simulink model "test_induction_cooker_increasedecreasepower"  (R2022b)
settings: Solver=FixedStepAuto  StartTime=0.0  StopTime=120  FixedStep=0.1  RelTol=1e-3
settings Model: Creator=cristian  LastModifiedBy=cristian
settings ConfigComp: CovEnable=on  CovScope=ReferencedModels  CovIncludeTopModel=off  CovModelRefEnable=filtered

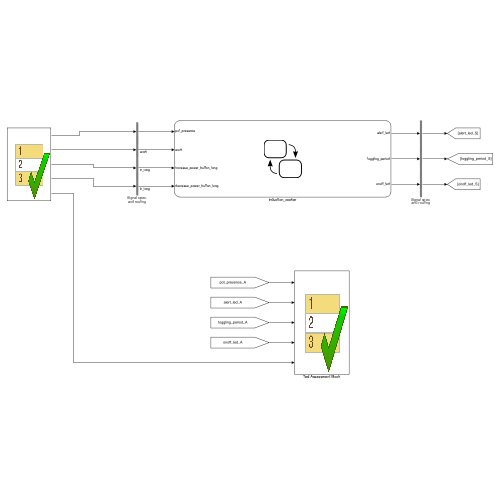
[thumbnail: Simulink's stored preview of the top-level diagram]
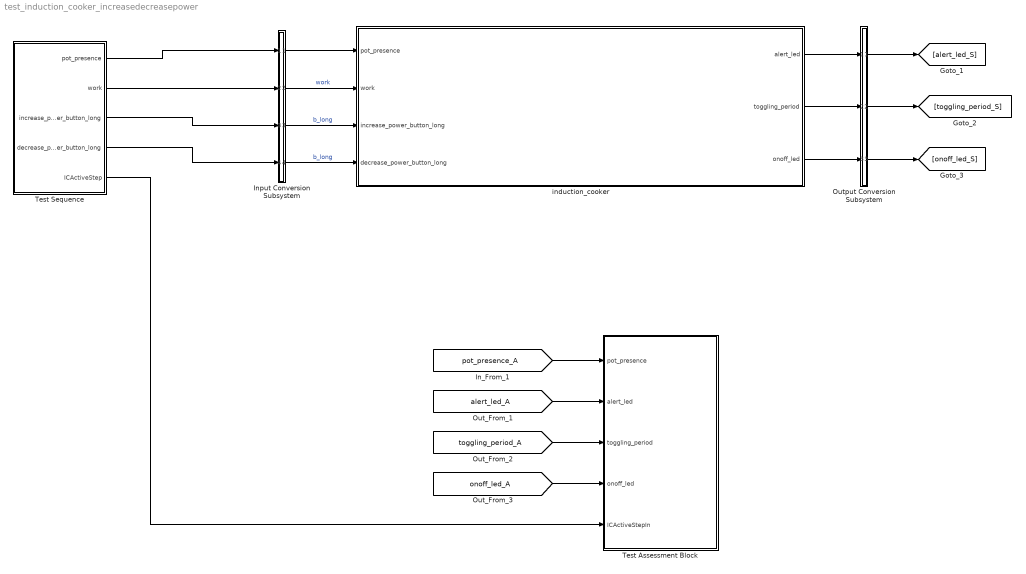
== system test_induction_cooker_increasedecreasepower ==
  Input Conversion Subsystem : Subsystem  Tag=__SLT_ICS__  Description=|
      | Signal spec.
      | and routing
      settings: AttributesFormatString=%<Description>
  Output Conversion Subsystem : Subsystem  Tag=__SLT_OCS__  Description=|
      | Signal spec.
      | and routing
      settings: AttributesFormatString=%<Description>
  Test Assessment Block : Test Sequence  Tag=__SLT_ASMT__  TreatAsAtomicUnit=on
  Test Sequence : Test Sequence  TreatAsAtomicUnit=on
  induction_cooker : Stateflow chart  TreatAsAtomicUnit=on
  wires:
  Test Sequence/1(pot_presence) -> Input Conversion Subsystem/1(Inport_1)
  Test Sequence/2(work) -> Input Conversion Subsystem/2(Inport_2)
  Test Sequence/3(increase_power_button_long) -> Input Conversion Subsystem/3(Inport_3)
  Test Sequence/4(decrease_power_button_long) -> Input Conversion Subsystem/4(Inport_4)
  Output Conversion Subsystem/1(Outport_1) -> [alert_led_S]
  Output Conversion Subsystem/2(Outport_2) -> [toggling_period_S]
  Output Conversion Subsystem/3(Outport_3) -> [onoff_led_S]
  Input Conversion Subsystem/1(Outport_1) -> induction_cooker/1(pot_presence)
  Input Conversion Subsystem/2(Outport_2) -> induction_cooker/2(work)  "work"
  Input Conversion Subsystem/3(Outport_3) -> induction_cooker/3(increase_power_button_long)  "b_long"
  Input Conversion Subsystem/4(Outport_4) -> induction_cooker/4(decrease_power_button_long)  "b_long"
  induction_cooker/1(alert_led) -> Output Conversion Subsystem/1(Inport_1)
  induction_cooker/2(toggling_period) -> Output Conversion Subsystem/2(Inport_2)
  induction_cooker/3(onoff_led) -> Output Conversion Subsystem/3(Inport_3)
  [onoff_led_A] -> Test Assessment Block/4(onoff_led)
  Test Sequence/5(ICActiveStep) -> Test Assessment Block/5(ICActiveStepIn)
  [toggling_period_A] -> Test Assessment Block/3(toggling_period)
  [alert_led_A] -> Test Assessment Block/2(alert_led)
  [pot_presence_A] -> Test Assessment Block/1(pot_presence)

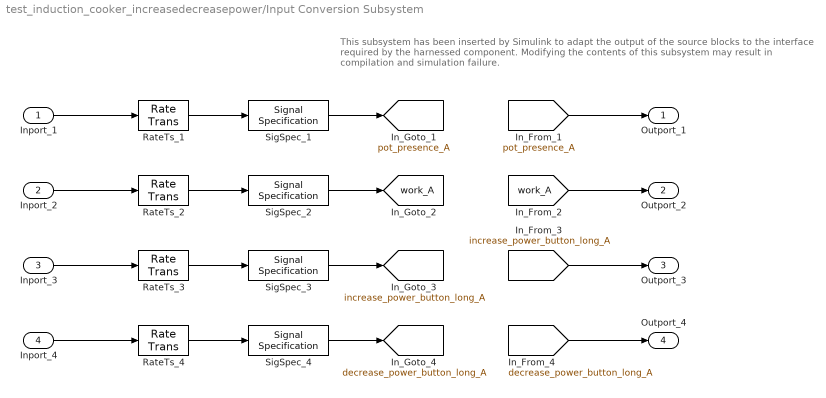
== system test_induction_cooker_increasedecreasepower/Input Conversion Subsystem ==
  note: This subsystem has been inserted by Simulink to adapt the output of the source blocks to the interface required by the harnessed component.
      |  Modifying the contents of this subsystem may result in compilation and simulation failure.
  Inport_1 : Inport
  Inport_2 : Inport  Port=2
  Inport_3 : Inport  Port=3
  Inport_4 : Inport  Port=4
  RateTs_1 : RateTransition  OutPortSampleTime=[-1, 0]
  RateTs_2 : RateTransition  OutPortSampleTime=[0, 1]
  RateTs_3 : RateTransition  OutPortSampleTime=[0, 1]
  RateTs_4 : RateTransition  OutPortSampleTime=[0, 1]
  SigSpec_1 : SignalSpecification  OutDataTypeStr=boolean  Dimensions=[1]  SampleTime=[-1, 0]
  SigSpec_2 : SignalSpecification  OutDataTypeStr=boolean  Dimensions=[1]  SampleTime=[0, 1]
  SigSpec_3 : SignalSpecification  OutDataTypeStr=boolean  Dimensions=[1]  SampleTime=[0, 1]
  SigSpec_4 : SignalSpecification  OutDataTypeStr=boolean  Dimensions=[1]  SampleTime=[0, 1]
  Outport_1 : Outport
  Outport_2 : Outport  Port=2
  Outport_3 : Outport  Port=3
  Outport_4 : Outport  Port=4
  tag scope: decrease_power_button_long_A=global, increase_power_button_long_A=global, pot_presence_A=global, work_A=global
  wires:
  [pot_presence_A] -> Outport_1/1
  SigSpec_1/1 -> [pot_presence_A]
  RateTs_1/1 -> SigSpec_1/1
  Inport_1/1 -> RateTs_1/1
  [work_A] -> Outport_2/1
  SigSpec_2/1 -> [work_A]
  RateTs_2/1 -> SigSpec_2/1
  Inport_2/1 -> RateTs_2/1
  [increase_power_button_long_A] -> Outport_3/1
  SigSpec_3/1 -> [increase_power_button_long_A]
  RateTs_3/1 -> SigSpec_3/1
  Inport_3/1 -> RateTs_3/1
  [decrease_power_button_long_A] -> Outport_4/1
  SigSpec_4/1 -> [decrease_power_button_long_A]
  RateTs_4/1 -> SigSpec_4/1
  Inport_4/1 -> RateTs_4/1

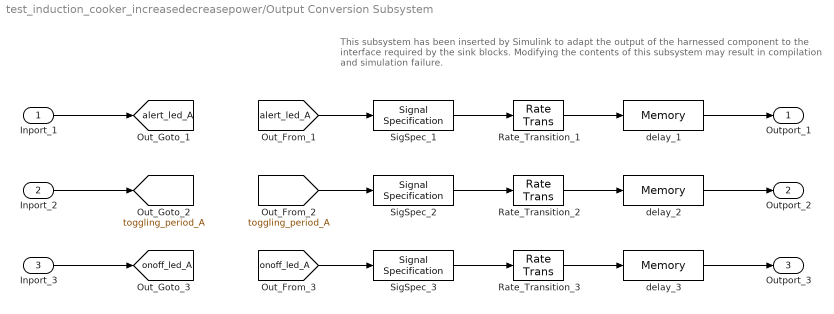
== system test_induction_cooker_increasedecreasepower/Output Conversion Subsystem ==
  note: This subsystem has been inserted by Simulink to adapt the output of the harnessed component to the interface required by the sink blocks.
      |  Modifying the contents of this subsystem may result in compilation and simulation failure.
  Inport_1 : Inport
  Inport_2 : Inport  Port=2
  Inport_3 : Inport  Port=3
  Rate_Transition_1 : RateTransition  OutPortSampleTimeOpt=Inherit
  Rate_Transition_2 : RateTransition  OutPortSampleTimeOpt=Inherit
  Rate_Transition_3 : RateTransition  OutPortSampleTimeOpt=Inherit
  SigSpec_1 : SignalSpecification  OutDataTypeStr=boolean  Dimensions=[1]
  SigSpec_2 : SignalSpecification  OutDataTypeStr=double  Dimensions=[1]
  SigSpec_3 : SignalSpecification  OutDataTypeStr=boolean  Dimensions=[1]
  delay_1 : Memory
  delay_2 : Memory
  delay_3 : Memory
  Outport_1 : Outport
  Outport_2 : Outport  Port=2
  Outport_3 : Outport  Port=3
  tag scope: alert_led_A=global, onoff_led_A=global, toggling_period_A=global
  wires:
  Inport_1/1 -> [alert_led_A]
  [alert_led_A] -> SigSpec_1/1
  SigSpec_1/1 -> Rate_Transition_1/1
  Rate_Transition_1/1 -> delay_1/1
  delay_1/1 -> Outport_1/1
  Inport_2/1 -> [toggling_period_A]
  [toggling_period_A] -> SigSpec_2/1
  SigSpec_2/1 -> Rate_Transition_2/1
  Rate_Transition_2/1 -> delay_2/1
  delay_2/1 -> Outport_2/1
  Inport_3/1 -> [onoff_led_A]
  [onoff_led_A] -> SigSpec_3/1
  SigSpec_3/1 -> Rate_Transition_3/1
  Rate_Transition_3/1 -> delay_3/1
  delay_3/1 -> Outport_3/1

== stateflow chart test_induction_cooker_increasedecreasepower/Test Assessment Block ==
  state IncreaseToMaxPower
    state step_1
      state Verify_IncreaseDecreasePower_Init
        verify(pot_presence == 0 && alert_led == 0 && abs(toggling_period - 0) < TOLERANCE && onoff_led == 0)
        settings: description=|
            | Inizializzazione.
            | Pentola presente, led di alert spento e potenza di erogazione nulla.
      state Verify_IncreaseDecreasePower_PowerOn
        verify(pot_presence == 0 && alert_led == 0 && abs(toggling_period - 0) < TOLERANCE && onoff_led == 1)
        settings: description=Richiesta di accensione del fornello.
      state Verify_IncreaseToMaxPower_PressFor300W
        verify(pot_presence == 0 && alert_led == 0 && abs(toggling_period - 0) < TOLERANCE && onoff_led == 1)
        settings: description=|
            | Pressione di richiesta incremento.
            | Pentola presente, led di alert spento e potenza di erogazione nulla.
            | Led di accensione acceso.
      state Verify_IncreaseToMaxPower_ReleaseFor300W
        verify(pot_presence == 0 && alert_led == 0 && abs(toggling_period - 0) < TOLERANCE && onoff_led == 1)
        settings: description=|
            | Rilascio bottone.
            | Pentola presente, led di alert spento e potenza di erogazione nulla.
            | Led di accensione acceso.
      state Verify_IncreaseToMaxPower_WaitIn300W
        verify(pot_presence == 0 && alert_led == 0 && abs(toggling_period - 2) < TOLERANCE && onoff_led == 1)
        settings: description=|
            | Stato di attesa di cambiamento potenza.
            | Pentola presente, led di alert spento e potenza di erogazione nulla.
            | Led di accensione acceso.
            | Frequenza di toggling incrementata.
      state Verify_IncreaseToMaxPower_PressFor500W
        verify(pot_presence == 0 && alert_led == 0 && abs(toggling_period - 2) < TOLERANCE && onoff_led == 1)
        settings: description=Pressione di richiesta incremento.
      state Verify_IncreaseToMaxPower_ReleaseFor500W
        verify(pot_presence == 0 && alert_led == 0 && abs(toggling_period - 2) < TOLERANCE && onoff_led == 1)
        settings: description=Rilascio bottone.
      state Verify_IncreaseToMaxPower_WaitIn500W
        verify(pot_presence == 0 && alert_led == 0 && abs(toggling_period - 1) < TOLERANCE && onoff_led == 1)
        settings: description=|
            | Stato di attesa di cambiamento potenza.
            | Pentola presente, led di alert spento e potenza di erogazione nulla.
            | Led di accensione acceso.
            | Frequenza di toggling incrementata.
      state Verify_IncreaseToMaxPower_PressFor1000W
        verify(pot_presence == 0 && alert_led == 0 && abs(toggling_period - 1) < TOLERANCE && onoff_led == 1)
        settings: description=Pressione di richiesta incremento.
      state Verify_IncreaseToMaxPower_ReleaseFor1000W
        verify(pot_presence == 0 && alert_led == 0 && abs(toggling_period - 1) < TOLERANCE && onoff_led == 1)
        settings: description=Rilascio bottone.
      state Verify_IncreaseToMaxPower_WaitIn1000W
        verify(pot_presence == 0 && alert_led == 0 && abs(toggling_period - 0.5) < TOLERANCE && onoff_led == 1)
        settings: description=|
            | Stato di attesa di cambiamento potenza.
            | Pentola presente, led di alert spento e potenza di erogazione nulla.
            | Led di accensione acceso.
            | Frequenza di toggling incrementata.
      state Verify_IncreaseToMaxPower_PressFor1500W
        verify(pot_presence == 0 && alert_led == 0 && abs(toggling_period - 0.5) < TOLERANCE && onoff_led == 1)
        settings: description=Pressione di richiesta incremento.
      state Verify_IncreaseToMaxPower_ReleaseFor1500W
        verify(pot_presence == 0 && alert_led == 0 && abs(toggling_period - 0.5) < TOLERANCE && onoff_led == 1)
        settings: description=Rilascio bottone.
      state Verify_IncreaseToMaxPower_WaitIn1500W
        verify(pot_presence == 0 && alert_led == 0 && abs(toggling_period - 0.25) < TOLERANCE && onoff_led == 1)
        settings: description=|
            | Stato di attesa di cambiamento potenza.
            | Pentola presente, led di alert spento e potenza di erogazione nulla.
            | Led di accensione acceso.
            | Frequenza di toggling incrementata.
      state Verify_DecreaseToMinPower_PressFor1000W
        verify(pot_presence == 0 && alert_led == 0 && abs(toggling_period - 0.25) < TOLERANCE && onoff_led == 1)
        settings: description=Pressione di richiesta decremento.
      state Verify_DecreaseToMinPower_ReleaseFor1000W
        verify(pot_presence == 0 && alert_led == 0 && abs(toggling_period - 0.25) < TOLERANCE && onoff_led == 1)
        settings: description=Rilascio bottone.
      state Verify_DecreaseToMinPower_WaitIn1000W
        verify(pot_presence == 0 && alert_led == 0 && abs(toggling_period - 0.50) < TOLERANCE && onoff_led == 1)
        settings: description=|
            | Stato di attesa di cambiamento potenza.
            | Pentola presente, led di alert spento e potenza di erogazione nulla.
            | Led di accensione acceso.
            | Frequenza di toggling decrementata.
      state Verify_DecreaseToMinPower_PressFor500W
        verify(pot_presence == 0 && alert_led == 0 && abs(toggling_period - 0.50) < TOLERANCE && onoff_led == 1)
        settings: description=Pressione di richiesta decremento.
      state Verify_DecreaseToMinPower_ReleaseFor500W
        verify(pot_presence == 0 && alert_led == 0 && abs(toggling_period - 0.50) < TOLERANCE && onoff_led == 1)
        settings: description=Rilascio bottone.
      state Verify_DecreaseToMinPower_WaitIn500W
        verify(pot_presence == 0 && alert_led == 0 && abs(toggling_period - 1) < TOLERANCE && onoff_led == 1)
        settings: description=|
            | Stato di attesa di cambiamento potenza.
            | Pentola presente, led di alert spento e potenza di erogazione nulla.
            | Led di accensione acceso.
            | Frequenza di toggling decrementata.
      state Verify_DecreaseToMinPower_PressFor300W
        verify(pot_presence == 0 && alert_led == 0 && abs(toggling_period - 1) < TOLERANCE && onoff_led == 1)
        settings: description=Pressione di richiesta decremento.
      state Verify_DecreaseToMinPower_ReleaseFor300W
        verify(pot_presence == 0 && alert_led == 0 && abs(toggling_period - 1) < TOLERANCE && onoff_led == 1)
        settings: description=Rilascio bottone.
      state Verify_DecreaseToMinPower_WaitIn300W
        verify(pot_presence == 0 && alert_led == 0 && abs(toggling_period - 2) < TOLERANCE && onoff_led == 1)
        settings: description=|
            | Stato di attesa di cambiamento potenza.
            | Pentola presente, led di alert spento e potenza di erogazione nulla.
            | Led di accensione acceso.
            | Frequenza di toggling decrementata.
      state step_1_1
      (default) -> (junction 238)
      step_1 -> (junction 238)
      (junction 238) -> (junction 239) [order 1] : [ICActiveStepIn == ICActiveStepEnum.IncreaseDecreasePower_Init
          | ]
      (junction 239) -> Verify_IncreaseDecreasePower_Init [order 1] : [~in(IncreaseToMaxPower.step_1.Verify_IncreaseDecreasePower_Init)]
      (junction 238) -> (junction 250) [order 2]
      (junction 239) -> (junction 242) [order 2]
      (junction 250) -> (junction 251) [order 1] : [ICActiveStepIn == ICActiveStepEnum.IncreaseDecreasePower_PowerOn
          | ]
      (junction 251) -> Verify_IncreaseDecreasePower_PowerOn [order 1] : [~in(IncreaseToMaxPower.step_1.Verify_IncreaseDecreasePower_PowerOn)]
      (junction 250) -> (junction 259) [order 2]
      (junction 251) -> (junction 254) [order 2]
      (junction 259) -> (junction 260) [order 1] : [ICActiveStepIn == ICActiveStepEnum.IncreaseToMaxPower_PressFor300W
          | ]
      (junction 260) -> Verify_IncreaseToMaxPower_PressFor300W [order 1] : [~in(IncreaseToMaxPower.step_1.Verify_IncreaseToMaxPower_PressFor300W)]
      (junction 259) -> (junction 268) [order 2]
      (junction 260) -> (junction 263) [order 2]
      (junction 268) -> (junction 269) [order 1] : [ICActiveStepIn == ICActiveStepEnum.IncreaseToMaxPower_ReleaseFor300W
          | ]
      (junction 269) -> Verify_IncreaseToMaxPower_ReleaseFor300W [order 1] : [~in(IncreaseToMaxPower.step_1.Verify_IncreaseToMaxPower_ReleaseFor300W)]
      (junction 268) -> (junction 277) [order 2]
      (junction 269) -> (junction 272) [order 2]
      (junction 277) -> (junction 278) [order 1] : [ICActiveStepIn == ICActiveStepEnum.IncreaseToMaxPower_WaitIn300W
          | ]
      (junction 278) -> Verify_IncreaseToMaxPower_WaitIn300W [order 1] : [~in(IncreaseToMaxPower.step_1.Verify_IncreaseToMaxPower_WaitIn300W)]
      (junction 277) -> (junction 286) [order 2]
      (junction 278) -> (junction 281) [order 2]
      (junction 286) -> (junction 287) [order 1] : [ICActiveStepIn == ICActiveStepEnum.IncreaseToMaxPower_PressFor500W
          | ]
      (junction 287) -> Verify_IncreaseToMaxPower_PressFor500W [order 1] : [~in(IncreaseToMaxPower.step_1.Verify_IncreaseToMaxPower_PressFor500W)]
      (junction 286) -> (junction 295) [order 2]
      (junction 287) -> (junction 290) [order 2]
      (junction 295) -> (junction 296) [order 1] : [ICActiveStepIn == ICActiveStepEnum.IncreaseToMaxPower_ReleaseFor500W
          | ]
      (junction 296) -> Verify_IncreaseToMaxPower_ReleaseFor500W [order 1] : [~in(IncreaseToMaxPower.step_1.Verify_IncreaseToMaxPower_ReleaseFor500W)]
      (junction 295) -> (junction 304) [order 2]
      (junction 296) -> (junction 299) [order 2]
      (junction 304) -> (junction 305) [order 1] : [ICActiveStepIn == ICActiveStepEnum.IncreaseToMaxPower_WaitIn500W
          | ]
      (junction 305) -> Verify_IncreaseToMaxPower_WaitIn500W [order 1] : [~in(IncreaseToMaxPower.step_1.Verify_IncreaseToMaxPower_WaitIn500W)]
      (junction 304) -> (junction 313) [order 2]
      (junction 305) -> (junction 308) [order 2]
      (junction 313) -> (junction 314) [order 1] : [ICActiveStepIn == ICActiveStepEnum.IncreaseToMaxPower_PressFor1000W
          | ]
      (junction 314) -> Verify_IncreaseToMaxPower_PressFor1000W [order 1] : [~in(IncreaseToMaxPower.step_1.Verify_IncreaseToMaxPower_PressFor1000W)]
      (junction 313) -> (junction 322) [order 2]
      (junction 314) -> (junction 317) [order 2]
      (junction 322) -> (junction 323) [order 1] : [ICActiveStepIn == ICActiveStepEnum.IncreaseToMaxPower_ReleaseFor1000W
          | ]
      (junction 323) -> Verify_IncreaseToMaxPower_ReleaseFor1000W [order 1] : [~in(IncreaseToMaxPower.step_1.Verify_IncreaseToMaxPower_ReleaseFor1000W)]
      (junction 322) -> (junction 331) [order 2]
      (junction 323) -> (junction 326) [order 2]
      (junction 331) -> (junction 332) [order 1] : [ICActiveStepIn == ICActiveStepEnum.IncreaseToMaxPower_WaitIn1000W
          | ]
      (junction 332) -> Verify_IncreaseToMaxPower_WaitIn1000W [order 1] : [~in(IncreaseToMaxPower.step_1.Verify_IncreaseToMaxPower_WaitIn1000W)]
      (junction 331) -> (junction 340) [order 2]
      (junction 332) -> (junction 335) [order 2]
      (junction 340) -> (junction 341) [order 1] : [ICActiveStepIn == ICActiveStepEnum.IncreaseToMaxPower_PressFor1500W
          | ]
      (junction 341) -> Verify_IncreaseToMaxPower_PressFor1500W [order 1] : [~in(IncreaseToMaxPower.step_1.Verify_IncreaseToMaxPower_PressFor1500W)]
      (junction 340) -> (junction 349) [order 2]
      (junction 341) -> (junction 344) [order 2]
      (junction 349) -> (junction 350) [order 1] : [ICActiveStepIn == ICActiveStepEnum.IncreaseToMaxPower_ReleaseFor1500W
          | ]
      (junction 350) -> Verify_IncreaseToMaxPower_ReleaseFor1500W [order 1] : [~in(IncreaseToMaxPower.step_1.Verify_IncreaseToMaxPower_ReleaseFor1500W)]
      (junction 349) -> (junction 358) [order 2]
      (junction 350) -> (junction 353) [order 2]
      (junction 358) -> (junction 359) [order 1] : [ICActiveStepIn == ICActiveStepEnum.IncreaseToMaxPower_WaitIn1500W
          | ]
      (junction 359) -> Verify_IncreaseToMaxPower_WaitIn1500W [order 1] : [~in(IncreaseToMaxPower.step_1.Verify_IncreaseToMaxPower_WaitIn1500W)]
      (junction 358) -> (junction 367) [order 2]
      (junction 359) -> (junction 362) [order 2]
      (junction 367) -> (junction 368) [order 1] : [ICActiveStepIn == ICActiveStepEnum.DecreaseToMinPower_PressFor1000W
          | ]
      (junction 368) -> Verify_DecreaseToMinPower_PressFor1000W [order 1] : [~in(IncreaseToMaxPower.step_1.Verify_DecreaseToMinPower_PressFor1000W)]
      (junction 367) -> (junction 376) [order 2]
      (junction 368) -> (junction 371) [order 2]
      (junction 376) -> (junction 377) [order 1] : [ICActiveStepIn == ICActiveStepEnum.DecreaseToMinPower_ReleaseFor1000W
          | ]
      (junction 377) -> Verify_DecreaseToMinPower_ReleaseFor1000W [order 1] : [~in(IncreaseToMaxPower.step_1.Verify_DecreaseToMinPower_ReleaseFor1000W)]
      (junction 376) -> (junction 385) [order 2]
      (junction 377) -> (junction 380) [order 2]
      (junction 385) -> (junction 386) [order 1] : [ICActiveStepIn == ICActiveStepEnum.DecreaseToMinPower_WaitIn1000W
          | ]
      (junction 386) -> Verify_DecreaseToMinPower_WaitIn1000W [order 1] : [~in(IncreaseToMaxPower.step_1.Verify_DecreaseToMinPower_WaitIn1000W)]
      (junction 385) -> (junction 394) [order 2]
      (junction 386) -> (junction 389) [order 2]
      (junction 394) -> (junction 395) [order 1] : [ICActiveStepIn == ICActiveStepEnum.DecreaseToMinPower_PressFor500W
          | ]
      (junction 395) -> Verify_DecreaseToMinPower_PressFor500W [order 1] : [~in(IncreaseToMaxPower.step_1.Verify_DecreaseToMinPower_PressFor500W)]
      (junction 394) -> (junction 403) [order 2]
      (junction 395) -> (junction 398) [order 2]
      (junction 403) -> (junction 404) [order 1] : [ICActiveStepIn == ICActiveStepEnum.DecreaseToMinPower_ReleaseFor500W
          | ]
      (junction 404) -> Verify_DecreaseToMinPower_ReleaseFor500W [order 1] : [~in(IncreaseToMaxPower.step_1.Verify_DecreaseToMinPower_ReleaseFor500W)]
      (junction 403) -> (junction 412) [order 2]
      (junction 404) -> (junction 407) [order 2]
      (junction 412) -> (junction 413) [order 1] : [ICActiveStepIn == ICActiveStepEnum.DecreaseToMinPower_WaitIn500W
          | ]
      (junction 413) -> Verify_DecreaseToMinPower_WaitIn500W [order 1] : [~in(IncreaseToMaxPower.step_1.Verify_DecreaseToMinPower_WaitIn500W)]
      (junction 412) -> (junction 421) [order 2]
      (junction 413) -> (junction 416) [order 2]
      (junction 421) -> (junction 422) [order 1] : [ICActiveStepIn == ICActiveStepEnum.DecreaseToMinPower_PressFor300W
          | ]
      (junction 422) -> Verify_DecreaseToMinPower_PressFor300W [order 1] : [~in(IncreaseToMaxPower.step_1.Verify_DecreaseToMinPower_PressFor300W)]
      (junction 421) -> (junction 430) [order 2]
      (junction 422) -> (junction 425) [order 2]
      (junction 430) -> (junction 431) [order 1] : [ICActiveStepIn == ICActiveStepEnum.DecreaseToMinPower_ReleaseFor300W
          | ]
      (junction 431) -> Verify_DecreaseToMinPower_ReleaseFor300W [order 1] : [~in(IncreaseToMaxPower.step_1.Verify_DecreaseToMinPower_ReleaseFor300W)]
      (junction 430) -> (junction 438) [order 2]
      (junction 431) -> (junction 434) [order 2]
      (junction 438) -> (junction 439) [order 1] : [ICActiveStepIn == ICActiveStepEnum.DecreaseToMinPower_WaitIn300W
          | ]
      (junction 439) -> Verify_DecreaseToMinPower_WaitIn300W [order 1] : [~in(IncreaseToMaxPower.step_1.Verify_DecreaseToMinPower_WaitIn300W)]
      (junction 438) -> (junction 446) [order 2]
      (junction 439) -> (junction 442) [order 2]
      (junction 446) -> (junction 447)
      (junction 447) -> step_1_1 [order 1] : [~in(IncreaseToMaxPower.step_1.step_1_1)]
      (junction 447) -> (junction 450) [order 2]
    (default) -> step_1
  (default) -> IncreaseToMaxPower : {assert(Active_Scenario_Index == 1,'The value of Scenario Parameter ''Active_Scenario_Index'' is not valid. Use the index of the scenario to specify it.')}
  data: pot_presence input boolean size=[1]; alert_led input boolean size=[1]; toggling_period input double size=[1]; onoff_led input boolean size=[1]; ICActiveStepIn input; Active_Scenario_Index parameter =1; TOLERANCE constant double =1e-9; sample_time constant double =str2num(get_param('InductionCooker','FixedStep'))

== stateflow chart test_induction_cooker_increasedecreasepower/induction_cooker ==
  note: Il core del fornello è composto da un chart principale che oscilla tra uno stato ON ed uno stato OFF, a seconda dell'input work che ne indica in che stato di funzionamento deve essere (associato al bottone a livelli di on/off).
  state OFF
    en: onoff_led = LOW, alert_led = LOW,
    current_power = 0, toggling_period = TOGGLING_PERIOD_OFF
  note: Lo stato ON è composto da tre macchine parallele che gestiscono rispettivamente: cambiamento potenza, allarme e blink del led.
  state ON
    state LOGIC [parallel]
      settings: executionOrder=1
      note: In LOGIC, lo stato di ingresso è quello a 0W, in quanto appena accendiamo il fornello esso non è attivo.
          | Quando si riceve l'input di INCREASE o DECREASE button, si transita in uno stato che rappresenta una nuova potenza selezionata, dopo 5 secondi da un passaggio di stato la potenza reale diventerà quella associata allo stato correntemente attivo.
          | Quando una certa potenza viene selezionata, viene aggiornato il periodo di blink del power_led.
      state P0W
        state WAIT
        state SET
          en:
          current_power = 0, toggling_period = TOGGLING_PERIOD_0W
        note: Lo stato che rappresenta 0W gode della particolarità di poter fissare la potenza anche senza attendere i 5s, questo è possibile quando da uno stato gerarchicamente superiore o parallelo viene impostato current_power = 0W. Tale circostanza avviene sia all'avvio in cui non vi è necessità di attendere del tempo prima di impostare la potenza a 0W e sia nel momento in cui scatta l'allarme, in cui si disattiva il fornello istantaneamente.
        (default) -> ON.LOGIC.P0W.WAIT
        ON.LOGIC.P0W.WAIT -> ON.LOGIC.P0W.SET : [after(SET_POWER_PATIENCE,sec) || current_power == 0]
      note: Notiamo che in ogni stato di LOGIC, diverso da 0W, vi è una transizione associata al fatto che la variabile alarm assume valore HIGH, che ci riporta automaticamente nello stato 0W e fissa tale potenza come potenza corrente senza attendere i 10 secondi.
      state P1500W
        state WAIT
        state SET
          en:
          current_power = 1500, toggling_period = TOGGLING_PERIOD_1500W
        (default) -> ON.LOGIC.P1500W.WAIT
        ON.LOGIC.P1500W.WAIT -> ON.LOGIC.P1500W.SET : after(SET_POWER_PATIENCE,sec)
      state P300W
        state WAIT
        state SET
          en:
          current_power = 300, toggling_period = TOGGLING_PERIOD_300W
        (default) -> ON.LOGIC.P300W.WAIT
        ON.LOGIC.P300W.WAIT -> ON.LOGIC.P300W.SET : after(SET_POWER_PATIENCE,sec)
      state P1000W
        state WAIT
        state SET
          en:
          current_power = 1000, toggling_period = TOGGLING_PERIOD_1000W
        (default) -> ON.LOGIC.P1000W.WAIT
        ON.LOGIC.P1000W.WAIT -> ON.LOGIC.P1000W.SET : after(SET_POWER_PATIENCE,sec)
      state P500W
        state WAIT
        state SET
          en:
          current_power = 500, toggling_period = TOGGLING_PERIOD_500W
        (default) -> ON.LOGIC.P500W.WAIT
        ON.LOGIC.P500W.WAIT -> ON.LOGIC.P500W.SET : after(SET_POWER_PATIENCE,sec)
      (default) -> P0W
      P1500W -> P0W [order 2] : [alarm == HIGH]
      P0W -> P300W : [increase_power_button_long == PRESSED && pot_presence == PRESSED]
      P300W -> P0W [order 1] : [(alarm == HIGH) || (decrease_power_button_long == PRESSED && pot_presence == PRESSED)]
      P500W -> P0W [order 3] : [alarm == HIGH]
      P1000W -> P0W [order 3] : [alarm == HIGH]
      P500W -> P300W [order 1] : [decrease_power_button_long == PRESSED && pot_presence == PRESSED]
      P300W -> P500W [order 2] : [increase_power_button_long == PRESSED && pot_presence == PRESSED]
      P1500W -> P1000W [order 1] : [decrease_power_button_long == PRESSED && pot_presence == PRESSED]
      P1000W -> P1500W [order 2] : [increase_power_button_long == PRESSED && pot_presence == PRESSED]
      P500W -> P1000W [order 2] : [increase_power_button_long == PRESSED && pot_presence == PRESSED]
      P1000W -> P500W [order 1] : [decrease_power_button_long == PRESSED && pot_presence == PRESSED]
    state TOGGLING_LED [parallel] [commented out]
      note: In ogni stato di LOGIC, che rappresenta una specifica potenza, viene impostato un valore di periodo che indica ogni quanto il power_led (led giallo) lampeggia.
          | Infatti, tale macchina semplicemente rimbalza da uno stato all'altro accendendo e spegnendo il led.
      state LED_OFF [commented out]
        en: power_led=LOW;
      state LED_ON [commented out]
        en: power_led=HIGH;
      (default) -> LED_OFF [commented out]
      LED_OFF -> LED_ON [commented out] : [toggling_period>0 && after(toggling_period,sec)]
      LED_ON -> LED_OFF [commented out] : [after(toggling_period,sec)]
    state ALARM [parallel]
      settings: executionOrder=2
      state ACTIVE
        state QUIET
          en: alarm = LOW, alert_led = LOW
        state ALARM
          en: alert_led = HIGH
          on after(ALARM_PATIENCE,sec): alarm = HIGH; current_power = 0; toggling_period = TOGGLING_PERIOD_0W; alert_led = LOW;
        (default) -> QUIET
        QUIET -> ON.ALARM.ACTIVE.ALARM : [pot_presence == RELEASED]
        ON.ALARM.ACTIVE.ALARM -> QUIET : [pot_presence == PRESSED]
      state INACTIVE
        en:
        alarm = LOW,
        alert_led = LOW
      (default) -> INACTIVE
      INACTIVE -> ACTIVE : [current_power ~= 0]
      ACTIVE -> INACTIVE : [current_power == 0]
  note: Quando la macchina non è attiva (current_power = 0W), anche l'allarme è inattivo. All'attivazione del fornello corrisponde l'attivazione dell'allarme.
      | Nel momento in cui l'allarme è attivo e rileva una rimozione della pentola passa in uno stato ALARM che accende l'alert_led e dopo 10 secondi di permanenza disattiva il sistema portando LOGIC nello stato 0W, a meno di reinserimento pentola che riporta in uno stato QUIET.
  (default) -> OFF
  OFF -> ON : [work == HIGH]{onoff_led = HIGH}
  ON -> OFF : [work == LOW]
  data: pot_presence input boolean size=1; work input boolean size=1; alarm local boolean size=1; alert_led output boolean size=1; toggling_period output double size=1; onoff_led output boolean size=1; current_power local uint16 size=1; increase_power_button_long input boolean size=1; decrease_power_button_long input boolean size=1; HIGH constant boolean size=1 =1; PRESSED constant boolean size=1 =0; RELEASED constant boolean size=1 =1; LOW constant boolean size=1 =0; ALARM_PATIENCE constant double =10; TOGGLING_PERIOD_0W constant double =0; TOGGLING_PERIOD_300W constant double =2; TOGGLING_PERIOD_500W constant double =1; TOGGLING_PERIOD_1000W constant double =0.5; TOGGLING_PERIOD_1500W constant double =0.25; SET_POWER_PATIENCE local =5; TOGGLING_PERIOD_OFF constant double =0

== stateflow chart test_induction_cooker_increasedecreasepower/Test Sequence ==
  settings: updateMethod=DISCRETE  sampleTime=0.1
  state IncreaseDecreasePower
    state IncreaseDecreasePower_Init
      pot_presence = false;
      work = false;
      increase_power_button_long = true;
      decrease_power_button_long = true;
      settings: description=|
          | Inizializzazione.
          | Inizialmente la pentola è presente, ed il dispositivo è acceso, ma non attivo.
          | E non è stato premuto il bottone che richiede la sua attivazione.
    state IncreaseDecreasePower_PowerOn
      work = true;
      settings: description=|
          | È stato premuto il bottone che richiede l'accensione del dispositivo.
          | La macchina viene accesa.
    state IncreaseToMaxPower
      settings: description=Di seguito richiediamo tutti i possibili livelli di incremento della potenza.
      state IncreaseToMaxPower_PressFor300W
        increase_power_button_long = false;
        settings: description=Viene premuto il pulsante per la richiesta di incremento della potenza.
      state IncreaseToMaxPower_ReleaseFor300W
        increase_power_button_long = true;
        settings: description=Il pulsante viene rilasciato.
      state IncreaseToMaxPower_WaitIn300W
        settings: description=Attesa della variazione di potenza.
      state IncreaseToMaxPower_PressFor500W
        increase_power_button_long = false;
        settings: description=Viene premuto il pulsante per la richiesta di incremento della potenza.
      state IncreaseToMaxPower_ReleaseFor500W
        increase_power_button_long = true;
        settings: description=Il pulsante viene rilasciato.
      state IncreaseToMaxPower_WaitIn500W
        settings: description=Attesa della variazione di potenza.
      state IncreaseToMaxPower_PressFor1000W
        increase_power_button_long = false;
        settings: description=Viene premuto il pulsante per la richiesta di incremento della potenza.
      state IncreaseToMaxPower_ReleaseFor1000W
        increase_power_button_long = true;
        settings: description=Il pulsante viene rilasciato.
      state IncreaseToMaxPower_WaitIn1000W
        settings: description=Attesa della variazione di potenza.
      state IncreaseToMaxPower_PressFor1500W
        increase_power_button_long = false;
        settings: description=Viene premuto il pulsante per la richiesta di incremento della potenza.
      state IncreaseToMaxPower_ReleaseFor1500W
        increase_power_button_long = true;
        settings: description=Il pulsante viene rilasciato.
      state IncreaseToMaxPower_WaitIn1500W
        settings: description=Attesa della variazione di potenza.
      (default) -> IncreaseToMaxPower_PressFor300W
      IncreaseToMaxPower_PressFor300W -> IncreaseToMaxPower_ReleaseFor300W : [
          | true
          | ]
      IncreaseToMaxPower_ReleaseFor300W -> IncreaseToMaxPower_WaitIn300W : [
          | after(5-sample_time,sec)
          | ]
      IncreaseToMaxPower_WaitIn300W -> IncreaseToMaxPower_PressFor500W : [
          | true
          | ]
      IncreaseToMaxPower_PressFor500W -> IncreaseToMaxPower_ReleaseFor500W : [
          | true
          | ]
      IncreaseToMaxPower_ReleaseFor500W -> IncreaseToMaxPower_WaitIn500W : [
          | after(5-sample_time,sec)
          | ]
      IncreaseToMaxPower_WaitIn500W -> IncreaseToMaxPower_PressFor1000W : [
          | true
          | ]
      IncreaseToMaxPower_PressFor1000W -> IncreaseToMaxPower_ReleaseFor1000W : [
          | true
          | ]
      IncreaseToMaxPower_ReleaseFor1000W -> IncreaseToMaxPower_WaitIn1000W : [
          | after(5-sample_time,sec)
          | ]
      IncreaseToMaxPower_WaitIn1000W -> IncreaseToMaxPower_PressFor1500W : [
          | true
          | ]
      IncreaseToMaxPower_PressFor1500W -> IncreaseToMaxPower_ReleaseFor1500W : [
          | true
          | ]
      IncreaseToMaxPower_ReleaseFor1500W -> IncreaseToMaxPower_WaitIn1500W : [
          | after(5-sample_time,sec)
          | ]
    state DecreaseToMinPower
      settings: description=Di seguito richiediamo tutti i possibili livelli di decremento della potenza.
      state DecreaseToMinPower_PressFor1000W
        decrease_power_button_long = false;
        settings: description=Viene premuto il pulsante per la richiesta di decremento della potenza.
      state DecreaseToMinPower_ReleaseFor1000W
        decrease_power_button_long = true;
        settings: description=Il pulsante viene rilasciato.
      state DecreaseToMinPower_WaitIn1000W
        settings: description=Attesa della variazione di potenza.
      state DecreaseToMinPower_PressFor500W
        decrease_power_button_long = false;
        settings: description=Viene premuto il pulsante per la richiesta di decremento della potenza.
      state DecreaseToMinPower_ReleaseFor500W
        decrease_power_button_long = true;
        settings: description=Il pulsante viene rilasciato.
      state DecreaseToMinPower_WaitIn500W
        settings: description=Attesa della variazione di potenza.
      state DecreaseToMinPower_PressFor300W
        decrease_power_button_long = false;
        settings: description=Viene premuto il pulsante per la richiesta di decremento della potenza.
      state DecreaseToMinPower_ReleaseFor300W
        decrease_power_button_long = true;
        settings: description=Il pulsante viene rilasciato.
      state DecreaseToMinPower_WaitIn300W
        settings: description=Attesa della variazione di potenza.
      (default) -> DecreaseToMinPower_PressFor1000W
      DecreaseToMinPower_PressFor1000W -> DecreaseToMinPower_ReleaseFor1000W : [
          | true
          | ]
      DecreaseToMinPower_WaitIn1000W -> DecreaseToMinPower_PressFor500W : [
          | true
          | ]
      DecreaseToMinPower_PressFor500W -> DecreaseToMinPower_ReleaseFor500W : [
          | true
          | ]
      DecreaseToMinPower_WaitIn500W -> DecreaseToMinPower_PressFor300W : [
          | true
          | ]
      DecreaseToMinPower_PressFor300W -> DecreaseToMinPower_ReleaseFor300W : [
          | true
          | ]
      DecreaseToMinPower_ReleaseFor1000W -> DecreaseToMinPower_WaitIn1000W : [
          | after(5-sample_time,sec)
          | ]
      DecreaseToMinPower_ReleaseFor500W -> DecreaseToMinPower_WaitIn500W : [
          | after(5-sample_time,sec)
          | ]
      DecreaseToMinPower_ReleaseFor300W -> DecreaseToMinPower_WaitIn300W : [
          | after(5-sample_time,sec)
          | ]
    (default) -> IncreaseDecreasePower_Init
    IncreaseDecreasePower_Init -> IncreaseDecreasePower_PowerOn : [
        | true
        | ]
    IncreaseDecreasePower_PowerOn -> IncreaseToMaxPower : [
        | after(2*sample_time,sec)
        | ]
    IncreaseToMaxPower -> DecreaseToMinPower : [
        | ICActiveStep == IncreaseToMaxPower_WaitIn1500W
        | ]
  (default) -> IncreaseDecreasePower : {assert(Active_Scenario_Index == 1,'The value of Scenario Parameter ''Active_Scenario_Index'' is not valid. Use the index of the scenario to specify it.')}
  data: pot_presence output boolean size=[1]; work output boolean size=[1]; increase_power_button_long output boolean size=[1]; decrease_power_button_long output boolean size=[1]; ICActiveStep output Enum: ICActiveStepEnum; Active_Scenario_Index parameter =1; sample_time constant double =str2num(get_param('InductionCooker','FixedStep'))
